simulink library "myLib"  (R2018a)
settings: Solver=VariableStepAuto  StartTime=0.0  StopTime=10.0  RelTol=1e-3
settings Model: Creator=Jason  LastModifiedBy=Jason

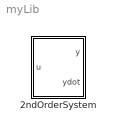
== system myLib ==
  2ndOrderSystem : Subsystem  mask{wn=1, zeta=0.707, p0=0, v0=0}
      mask prompts: wn "Natural Frequency (rad/s)"; zeta "Damping ratio"; p0 "Initial Position"; v0 "Initial Velocity"

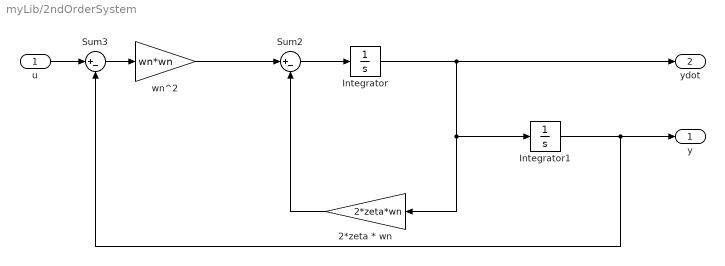
== system myLib/2ndOrderSystem ==
  u : Inport
  2*zeta * wn : Gain  Gain=2*zeta*wn  SaturateOnIntegerOverflow=on  OutDataTypeStr=Inherit: Same as input  ParamDataTypeStr=Inherit: Same as input
  Integrator : Integrator  InitialCondition=v0
  Integrator1 : Integrator  InitialCondition=p0
  Sum2 : Sum  Inputs=|+-  SaturateOnIntegerOverflow=on  InputSameDT=on  OutDataTypeStr=Inherit: Same as first input
  Sum3 : Sum  Inputs=|+-  SaturateOnIntegerOverflow=on  InputSameDT=on  OutDataTypeStr=Inherit: Same as first input
  wn^2 : Gain  Gain=wn*wn  SaturateOnIntegerOverflow=on  OutDataTypeStr=Inherit: Same as input  ParamDataTypeStr=Inherit: Same as input
  y : Outport  InitialOutput=0
  ydot : Outport  Port=2  InitialOutput=0
  wires:
  wn^2/1 -> Sum2/1
  Sum2/1 -> Integrator/1
  Integrator/1 -> Integrator1/1, 2*zeta * wn/1, ydot/1
  2*zeta * wn/1 -> Sum2/2
  Sum3/1 -> wn^2/1
  Integrator1/1 -> y/1, Sum3/2
  u/1 -> Sum3/1
